simulink model "BimanualHD2LfD"  (Simulink 8.8)
settings: Solver=ode1  StartTime=0.0  StopTime=inf  FixedStep=0.002  RelTol=1e-3  EnableMultiTasking=on
undefined symbols (not defined in the file or in its folder): d2r, HIL, qc_get_step_size
libraries: quarc_library x10, simulink_extras x4, dsparch4 x3, simulink x1
(part 2 of 2)

== matlab function HD2 Dynamics/Endonesial I//O/HD^2 New Kin new frame/New Numerical Kin ==
  data: q input double; pos output double; or output double; ang output double; poses output double; Trans output double; nn output double; x output double
 function [pos, or ,ang , poses, Trans, nn, x] = HDsquared_forwardkin(q)

    x = [0 0 0 0]';
    l = [220 40 125 22.25 250];
    ang = [0 0 0];
    
  
    nn = 0;
    while ( (norm(fnum(q,x,l)) > 0.0001) && nn <20)
      nn = nn+1;
        x = x - inv(Jnum(q,x,l))*fnum(q,x,l)';
    end
    
    
    
    pos = handlePos(q,x,l)';
    or = handleOr(q,x,l);
     
%     yaw = atan2 (or(2,1),or(1,1));   %AA
%     roll = atan2 ( or(3,2),or(3,3) );  %AA
%     pitch = atan2( -or(3,1), sqrt(  or(3,2)^2 + or(3,3)^2 ) ); %AA
%     
%     ang = [yaw;pitch;roll];  %AA
    
    pos_top = 250/2*(or(:,3))+pos;
    pos_bottom = -250/2*(or(:,3))+pos;
    poses = [pos_top;pos_bottom];
    
    Trans1 = cat(2,or,pos);
    Trans = cat(1,Trans1,[0 0 0 1]);
    
end


function val = fnum(q,x,l)

val = zeros(1,4); %AA
    q1 = q(1);
    q2 = q(2);
    q3 = q(3);
    q4 = q(4);
    q5 = q(5);
    q6 = q(6);
    
    l1 = l(1);
    l2 = l(2);
    l3 = l(3);
    l4 = l(4);
    l5 = l(5);
    
    alpha_u = x(1);
    theta_u = x(2);
    alpha_l = x(3);
    theta_l = x(4);
    
    t1 = pi / 0.4e1;
    t3 = cos(t1 + q1);
    t4 = sin(alpha_u);
    t5 = t3 * t4;
    t7 = cos(-t1 + q1);
    t8 = sin(theta_u);
    t9 = t7 * t8;
    t10 = cos(alpha_u);
    t11 = t9 * t10;
    t13 = cos(t1 + q4);
    t14 = sin(alpha_l);
    t15 = t13 * t14;
    t17 = cos(-t1 + q4);
    t18 = sin(theta_l);
    t19 = t17 * t18;
    t20 = cos(alpha_l);
    t21 = t19 * t20;
    t23 = cos(q3);
    t24 = t23 * t7;
    t25 = t24 * t4;
    t28 = sin(q3);
    t29 = cos(theta_u);
    t31 = t23 * t3 * t8 + t28 * t29;
    t32 = t31 * t10;
    t33 = cos(q6);
    t34 = t33 * t17;
    t35 = t34 * t14;
    t38 = sin(q6);
    t39 = cos(theta_l);
    t41 = t33 * t13 * t18 + t38 * t39;
    t42 = t41 * t20;
    t45 = cos(-t1 + q2);
    t56 = cos(-t1 + q5);
    t68 = cos(t1 + q2);
    t80 = cos(t1 + q5);
    val(1) = t5 + t11 - t15 - t21;
    val(2) = -t25 + t32 + t35 - t42;
    val(3) = t45 * l1 - t3 * l1 + (-t3 * t10 + t9 * t4) * l4 - (t5 + t11) * l5 / 0.2e1 - t56 * l1 + t13 * l1 - (-t13 * t20 + t19 * t14) * l4 - (t15 + t21) * l5 / 0.2e1;
    val(4) = t23 * t68 * l1 + t24 * l1 + (t24 * t10 + t31 * t4) * l4 - (-t25 + t32) * l5 / 0.2e1 - t33 * t80 * l1 - t34 * l1 - (t34 * t20 + t41 * t14) * l4 - (-t35 + t42) * l5 / 0.2e1;

end



function val2 = Jnum(q,x,l)
val2 = zeros(4,4); %AA
    q1 = q(1);
    q2 = q(2);
    q3 = q(3);
    q4 = q(4);
    q5 = q(5);
    q6 = q(6);
    
    l1 = l(1);
    l2 = l(2);
    l3 = l(3);
    l4 = l(4);
    l5 = l(5);
    
    
    alpha_u = x(1);
    theta_u = x(2);
    alpha_l = x(3);
    theta_l = x(4);
    
    t1 = pi / 0.4e1;
    t3 = cos(t1 + q1);
    t4 = cos(alpha_u);
    t7 = cos(-t1 + q1);
    t8 = sin(theta_u);
    t9 = t7 * t8;
    t10 = sin(alpha_u);
    t12 = t3 * t4 - t9 * t10;
    t13 = cos(theta_u);
    t14 = t7 * t13;
    t17 = cos(t1 + q4);
    t18 = cos(alpha_l);
    t21 = cos(-t1 + q4);
    t22 = sin(theta_l);
    t23 = t21 * t22;
    t24 = sin(alpha_l);
    t26 = -t17 * t18 + t23 * t24;
    t27 = cos(theta_l);
    t28 = t21 * t27;
    t30 = cos(q3);
    t31 = t30 * t7;
    t33 = t30 * t3;
    t35 = sin(q3);
    t37 = t33 * t8 + t35 * t13;
    t39 = -t31 * t4 - t37 * t10;
    t42 = t33 * t13 - t35 * t8;
    t43 = t42 * t4;
    t44 = cos(q6);
    t45 = t44 * t21;
    t47 = t44 * t17;
    t49 = sin(q6);
    t51 = t47 * t22 + t49 * t27;
    t53 = t45 * t18 + t51 * t24;
    t56 = t47 * t27 - t49 * t22;
    t57 = t56 * t18;
    val2(1,1) = t12;
    val2(1,2) = t14 * t4;
    val2(1,3) = t26;
    val2(1,4) = -t28 * t18;
    val2(2,1) = t39;
    val2(2,2) = t43;
    val2(2,3) = t53;
    val2(2,4) = -t57;
    val2(3,1) = (t3 * t10 + t9 * t4) * l4 - t12 * l5 / 0.2e1;
    val2(3,2) = t14 * t10 * l4 - t14 * t4 * l5 / 0.2e1;
    val2(3,3) = -(t17 * t24 + t23 * t18) * l4 + t26 * l5 / 0.2e1;
    val2(3,4) = -t28 * t24 * l4 - t28 * t18 * l5 / 0.2e1;
    val2(4,1) = (-t31 * t10 + t37 * t4) * l4 - t39 * l5 / 0.2e1;
    val2(4,2) = t42 * t10 * l4 - t43 * l5 / 0.2e1;
    val2(4,3) = -(-t45 * t24 + t51 * t18) * l4 + t53 * l5 / 0.2e1;
    val2(4,4) = -t56 * t24 * l4 - t57 * l5 / 0.2e1;

end

function val3 = handlePos(q,x,l)
 val3 = zeros(1,3);   %AA
    q1 = q(1);
    q2 = q(2);
    q3 = q(3);
    q4 = q(4);
    q5 = q(5);
    q6 = q(6);
    
    l1 = l(1);
    l2 = l(2);
    l3 = l(3);
    l4 = l(4);
    l5 = l(5);
    
    
    alpha_u = x(1);
    theta_u = x(2);
    alpha_l = x(3);
    theta_l = x(4);

    t1 = pi / 0.4e1;
    t3 = cos(-t1 + q2);
    t6 = cos(t1 + q1);
    t8 = cos(alpha_u);
    t11 = cos(-t1 + q1);
    t12 = sin(theta_u);
    t13 = t11 * t12;
    t14 = sin(alpha_u);
    t24 = cos(q3);
    t26 = cos(t1 + q2);
    t29 = t24 * t11;
    t34 = sin(q3);
    t35 = cos(theta_u);
    t37 = t24 * t6 * t12 + t34 * t35;
    t49 = t34 * t11;
    t55 = -t34 * t6 * t12 + t24 * t35;
    val3(1) = t3 * l1 - t6 * l1 + (-t6 * t8 + t13 * t14) * l4 - (t6 * t14 + t13 * t8) * l5 / 0.2e1;
    val3(2) = t24 * t26 * l1 + t29 * l1 + (t29 * t8 + t37 * t14) * l4 - (-t29 * t14 + t37 * t8) * l5 / 0.2e1;
    val3(3) = l3 - t34 * t26 * l1 - t49 * l1 + (-t49 * t8 + t55 * t14) * l4 - (t49 * t14 + t55 * t8) * l5 / 0.2e1;

end

function val4 = handleOr(q,x,l)
  val4 = zeros(3,3);  %AA 
    q1 = q(1);
    q2 = q(2);
    q3 = q(3);
    q4 = q(4);
    q5 = q(5);
    q6 = q(6);
    q7 = q(7);
    
    l1 = l(1);
    l2 = l(2);
    l3 = l(3);
    l4 = l(4);
    l5 = l(5);
    
    
    alpha_u = x(1);
    theta_u = x(2);
    alpha_l = x(3);
    theta_l = x(4);
    
    t1 = pi / 0.4e1;
    t3 = cos(-t1 + q1);
    t4 = cos(theta_u);
    t5 = t3 * t4;
    t6 = cos(q7);
    t9 = cos(t1 + q1);
    t10 = cos(alpha_u);
    t12 = sin(theta_u);
    t13 = t3 * t12;
    t14 = sin(alpha_u);
    t16 = -t9 * t10 + t13 * t14;
    t17 = sin(q7);
    t26 = cos(q3);
    t27 = t26 * t9;
    t29 = sin(q3);
    t31 = t27 * t4 - t29 * t12;
    t33 = t26 * t3;
    t37 = t27 * t12 + t29 * t4;
    t39 = t33 * t10 + t37 * t14;
    t48 = t29 * t9;
    t51 = -t48 * t4 - t26 * t12;
    t53 = t29 * t3;
    t57 = -t48 * t12 + t26 * t4;
    t59 = -t53 * t10 + t57 * t14;
    val4(1,1) = t5 * t6 + t16 * t17;
    val4(1,2) = -t5 * t17 + t16 * t6;
    val4(1,3) = t9 * t14 + t13 * t10;
    val4(2,1) = t31 * t6 + t39 * t17;
    val4(2,2) = -t31 * t17 + t39 * t6;
    val4(2,3) = -t33 * t14 + t37 * t10;
    val4(3,1) = t51 * t6 + t59 * t17;
    val4(3,2) = -t51 * t17 + t59 * t6;
    val4(3,3) = t53 * t14 + t57 * t10;

end

== matlab function HD2 Dynamics/Endonesial I//O/HIL Interfacing/Subsystem1/De Bouncer/Embedded MATLAB Function ==
  data: input input double; num_samples input int32; output output double; prev_output input double; prev_counter input int32; counter output int32
function [output, counter] = de_bouncer(input,  num_samples,prev_output, prev_counter)
if (prev_output ~= input)
    % Change detected
    counter = prev_counter - 1;
    if (counter == 0)
        output = input;
    else
        output = prev_output;
    end
else
    counter = num_samples;
    output = prev_output;
end

== matlab function HD2 Dynamics/Endonesial I//O/HIL Interfacing/Subsystem1/De Bouncer1/Embedded MATLAB Function ==
  data: input input double; num_samples input int32; output output double; prev_output input double; prev_counter input int32; counter output int32
function [output, counter] = de_bouncer(input,  num_samples,prev_output, prev_counter)
if (prev_output ~= input)
    % Change detected
    counter = prev_counter - 1;
    if (counter == 0)
        output = input;
    else
        output = prev_output;
    end
else
    counter = num_samples;
    output = prev_output;
end

== matlab function HD2 Dynamics/Endonesial I//O/Torque to Force ==
  data: x_lower input double; F_upper output double; F_lower output double; x_upper input double; tau input double; l11 input double; l22 input double
function [F_upper,F_lower] = fcn(x_lower,x_upper,tau,l11,l22)
% This block supports the Embedded MATLAB subset.
% See the help menu for details. 


%Initialization
F_upper=zeros(3,1);
F_lower=zeros(3,1);

if l11 == 0 
    sg1 = 1;
else
    sg1= sign(l11);
end

if l22 == 0 
    sg2 = 1;
else
    sg2= sign(l22);
end



if abs(l11)<0.005 
    l1 = 0.005 * sg1;
else
    l1= l11;
end

if abs(l22)<0.005 
    l2 = 0.005 * sg2;
else
    l2= l22;
end
%%%%%%%%%%%%%%%%%%%%%%%%%%%%

link = sqrt (  (x_upper(3)-x_lower(3))^2 + (x_upper(1)-x_lower(1))^2  + (x_upper(2)-x_lower(2))^2  );
unitvec = (x_upper - x_lower)/link;
F_upper = ( cross (tau,unitvec))/2/l1;
F_lower = - ( cross (tau,unitvec))/2/l2;


% link = sqrt (  (x_upper(3)-x_lower(3))^2 + (x_upper(1)-x_lower(1))^2  + (x_upper(2)-x_lower(2))^2  );
% unitvec = (x_upper - x_lower)/link;
% F_upper = 2/link * ( cross (tau,unitvec));
% F_lower = - F_upper;
% 

% link = sqrt (  (x_upper(3)-x_lower(3))^2 + (x_upper(1)-x_lower(1))^2  + (x_upper(2)-x_lower(2))^2  );
% unitvec = (x_lower - x_upper)/link;
% F_upper = (5/link * ( cross (tau,unitvec)));
% F_lower = F_upper/6;

== matlab function HD2 Dynamics/Endonesial I//O/Calculate Mean Position ==
  data: x_mean output double; x input double; l1 input double
function x_mean  = mean1(x,l1)
% This block supports the Embedded MATLAB subset.
% See the help menu for details. 
% link = .175;%25;
% l2=link - l1;
% 
% x_mean=zeros(3,1);
% x_mean(1)=(l2*x(1)+l1*x(4))/link;
% x_mean(2)=(l2*x(2)+l1*x(5))/link;
% x_mean(3)=(l2*x(3)+l1*x(6))/link;

x_mean=zeros(3,1);
x_mean(1)=(x(1)+x(4))/2;
x_mean(2)=(x(2)+x(5))/2;
x_mean(3)=(x(3)+x(6))/2;
